simulink model "sampleModel1925"  (R2023a)
settings: Solver=VariableStepAuto  StartTime=0.0  StopTime=10.0  RelTol=1e-3
libraries: simulink x6, hdlsllib x4
settings Model: Creator=user1  LastModifiedBy=user1

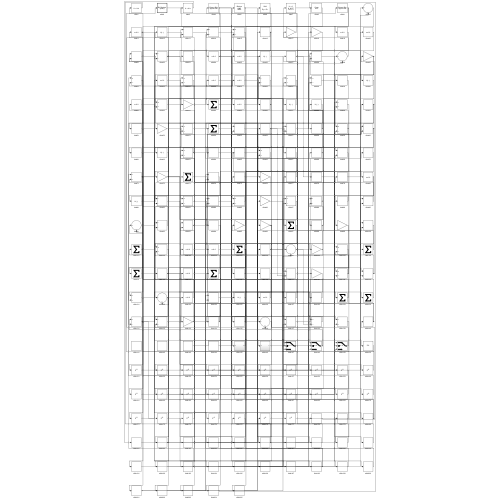
[thumbnail: Simulink's stored preview of the top-level diagram]
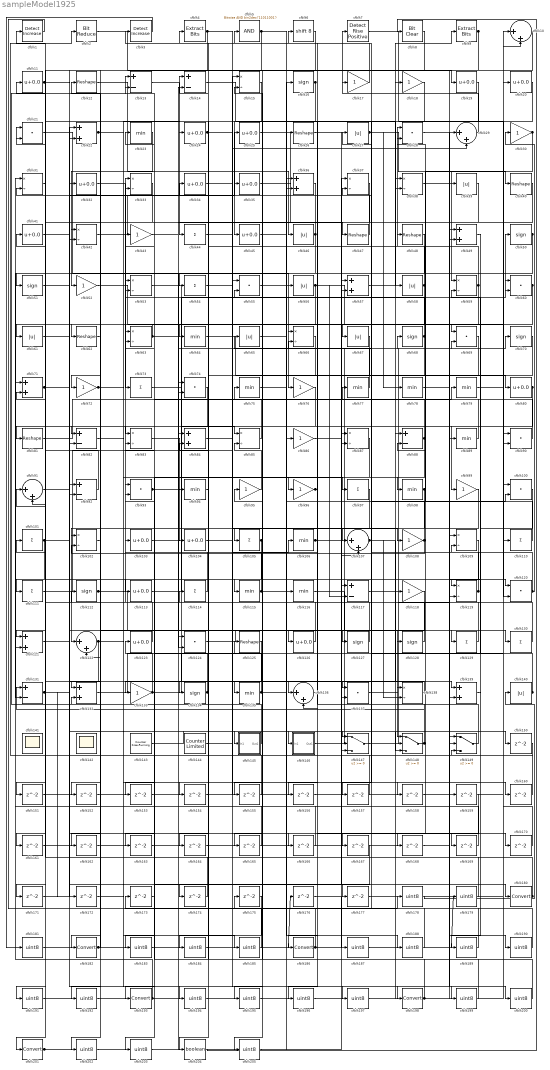
== system sampleModel1925 ==
  cfblk1 : simulink/Logic and Bit Operations/Detect Increase  vinit=0.0  OutDataTypeStr=boolean
      settings: LibrarySourceBlock=|
      | hdlsllib/Logic and Bit
      | Operations/Detect
      | Increase
  cfblk{10,29,91,107,122,136} (6 alike) : Sum  Inputs=|++
  cfblk{21,28,55,60,69,74,90,93,100,120,124,137} (12 alike) : DotProduct  OutDataTypeStr=Inherit: Inherit via internal rule
  cfblk{44,54,73,97,101,105,110..111,114,129..130} (11 alike) : Sum  Inputs=+
  cfblk{15,31,33,37..38,42,53,59,63,66,83,85,87,102,109,119,138} (17 alike) : Product  Inputs=*/  RndMeth=Zero  SaturateOnIntegerOverflow=on
  cfblk{11,19..20,24..25,32,34..35,41,45,80,103..104,113,123,126} (16 alike) : Bias  Bias=0.0  SaturateOnIntegerOverflow=off
  cfblk{23,64,75,77..79,89,94,98,106,115..116,135} (13 alike) : MinMax
  cfblk{17..18,30,43,52,72,76,86,95..96,99,108,118,133} (14 alike) : Gain
  cfblk{16,50..51,68,70,112,127..128,134} (9 alike) : Signum
  cfblk{13..14,82,88,92,117,131} (7 alike) : Sum  Inputs=+-
  cfblk{12,26,40,47..48,62,81,125} (8 alike) : Reshape
  cfblk{22,36,49,57,71,84,121,132,139} (9 alike) : Sum
  cfblk{27,39,46,56,58,61,65,67,140} (9 alike) : Abs  SaturateOnIntegerOverflow=off
  cfblk141 : Scope
      settings: Floating=on
  cfblk142 : Scope
      settings: Floating=on
  cfblk143 : hdlsllib/Sources/Counter Free-Running  NumBits=16  tsamp=-1
  cfblk144 : hdlsllib/Sources/Counter Limited  uplimit=7  tsamp=-1
  cfblk145 : Subsystem
      settings: LibrarySourceBlock=|
      | hdlsllib/Ports &
      | Subsystems/Subsystem
  cfblk146 : Subsystem
      settings: LibrarySourceBlock=|
      | hdlsllib/Ports &
      | Subsystems/Subsystem
  cfblk147 : Switch  SaturateOnIntegerOverflow=off  InputSameDT=off
  cfblk148 : Switch  SaturateOnIntegerOverflow=off  InputSameDT=off
  cfblk149 : Switch  SaturateOnIntegerOverflow=off  InputSameDT=off
  cfblk{150..177} (28 alike) : Delay  SampleTime=1
  cfblk{178..179,181,183..185,187..192,194..197,199..200,202..203,205} (21 alike) : DataTypeConversion  OutDataTypeStr=uint8  SaturateOnIntegerOverflow=off  RndMeth=Floor
  cfblk{180,182,186,193,198,201} (6 alike) : DataTypeConversion  SaturateOnIntegerOverflow=off  RndMeth=Floor
  cfblk2 : hdlsllib/Logic and Bit Operations/Bit Reduce  mode=AND
  cfblk204 : DataTypeConversion  OutDataTypeStr=boolean  SaturateOnIntegerOverflow=off  RndMeth=Floor
  cfblk3 : simulink/Logic and Bit Operations/Detect Increase  vinit=0.0  OutDataTypeStr=boolean
      settings: LibrarySourceBlock=|
      | hdlsllib/Logic and Bit
      | Operations/Detect
      | Increase
  cfblk4 : simulink/Logic and Bit Operations/Extract Bits  bitsToExtract=Upper half  numBits=8  bitIdxRange=[0 7]  outScalingMode=Preserve fixed-point scaling
      settings: LibrarySourceBlock=|
      | hdlsllib/Logic and Bit
      | Operations/Extract Bits
  cfblk5 : simulink/Logic and Bit Operations/Bitwise Operator  logicop=AND  UseBitMask=on  BitMask=bin2dec('11011001')  BitMaskRealWorld=Stored Integer
      settings: LibrarySourceBlock=|
      | hdlsllib/Logic and Bit
      | Operations/Bitwise
      | Operator
  cfblk6 : ArithShift  BitShiftNumber=8
  cfblk7 : hdlsllib/Logic and Bit Operations/Detect Rise Positive  vinit=0  OutDataTypeStr=boolean
  cfblk8 : simulink/Logic and Bit Operations/Bit Clear  iBit=0
      settings: LibrarySourceBlock=|
      | hdlsllib/Logic and Bit
      | Operations/Bit Clear
  cfblk9 : simulink/Logic and Bit Operations/Extract Bits  bitsToExtract=Upper half  numBits=8  bitIdxRange=[0 7]  outScalingMode=Preserve fixed-point scaling
      settings: LibrarySourceBlock=|
      | hdlsllib/Logic and Bit
      | Operations/Extract Bits
  wires:
  cfblk149/1 -> cfblk5/1
  cfblk53/1 -> cfblk85/1
  cfblk87/1 -> cfblk193/1
  cfblk146/1(Out1) -> cfblk68/1
  cfblk138/1 -> cfblk135/1
  cfblk23/1 -> cfblk52/1
  cfblk103/1 -> cfblk127/1
  cfblk11/1 -> cfblk170/1, cfblk171/1
  cfblk97/1 -> cfblk122/1
  cfblk81/1 -> cfblk79/1
  cfblk29/1 -> cfblk7/1
  cfblk129/1 -> cfblk33/1
  cfblk143/1 -> cfblk145/1(In1)
  cfblk88/1 -> cfblk96/1, cfblk53/2
  cfblk140/1 -> cfblk77/1, cfblk59/2
  cfblk26/1 -> cfblk180/1
  cfblk21/1 -> cfblk76/1
  cfblk106/1 -> cfblk37/1, cfblk138/1
  cfblk46/1 -> cfblk54/1, cfblk42/1
  cfblk147/1 -> cfblk70/1
  cfblk145/1(Out1) -> cfblk13/1
  cfblk116/1 -> cfblk148/1
  cfblk12/1 -> cfblk46/1
  cfblk73/1 -> cfblk137/1
  cfblk101/1 -> cfblk41/1, cfblk35/1, cfblk131/2
  cfblk32/1 -> cfblk73/1
  cfblk15/1 -> cfblk45/1
  cfblk64/1 -> cfblk109/1
  cfblk40/1 -> cfblk62/1
  cfblk65/1 -> cfblk116/1
  cfblk69/1 -> cfblk115/1
  cfblk58/1 -> cfblk28/1, cfblk102/1, cfblk27/1
  cfblk84/1 -> cfblk198/1
  cfblk102/1 -> cfblk122/2
  cfblk7/1 -> cfblk110/1
  cfblk108/1 -> cfblk37/2, cfblk102/2
  cfblk114/1 -> cfblk93/1
  cfblk89/1 -> cfblk63/1
  cfblk13/1 -> cfblk44/1
  cfblk139/1 -> cfblk2/1
  cfblk30/1 -> cfblk59/1, cfblk168/1
  cfblk85/1 -> cfblk13/2
  cfblk2/1 -> cfblk19/1
  cfblk61/1 -> cfblk147/1
  cfblk27/1 -> cfblk40/1, cfblk78/1
  cfblk48/1 -> cfblk124/2
  cfblk36/1 -> cfblk72/1
  cfblk42/1 -> cfblk25/1
  cfblk90/1 -> cfblk48/1
  cfblk113/1 -> cfblk50/1
  cfblk83/1 -> cfblk104/1
  cfblk115/1 -> cfblk14/1, cfblk100/2
  cfblk16/1 -> cfblk82/1, cfblk164/1
  cfblk111/1 -> cfblk15/1
  cfblk96/1 -> cfblk126/1, cfblk136/2
  cfblk118/1 -> cfblk182/1
  cfblk123/1 -> cfblk112/1
  cfblk39/1 -> cfblk98/1
  cfblk76/1 -> cfblk82/2
  cfblk6/1 -> cfblk105/1
  cfblk25/1 -> cfblk117/1
  cfblk131/1 -> cfblk136/1, cfblk172/1
  cfblk24/1 -> cfblk29/2, cfblk139/2
  cfblk17/1 -> cfblk3/1
  cfblk144/1 -> cfblk106/1
  cfblk59/1 -> cfblk111/1, cfblk4/1
  cfblk133/1 -> cfblk123/1, cfblk89/1
  cfblk105/1 -> cfblk151/1, cfblk152/1, cfblk195/1
  cfblk119/1 -> cfblk6/1, cfblk66/2
  cfblk4/1 -> cfblk108/1, cfblk22/2, cfblk167/1
  cfblk56/1 -> cfblk69/1, cfblk117/2, cfblk92/2
  cfblk28/1 -> cfblk130/1
  cfblk112/1 -> cfblk147/2, cfblk174/1
  cfblk50/1 -> cfblk132/1, cfblk121/2
  cfblk122/1 -> cfblk160/1, cfblk161/1
  cfblk93/1 -> cfblk39/1, cfblk53/1
  cfblk132/1 -> cfblk90/2
  cfblk47/1 -> cfblk31/2
  cfblk134/1 -> cfblk63/2, cfblk133/1
  cfblk37/1 -> cfblk147/3
  cfblk95/1 -> cfblk85/2
  cfblk60/1 -> cfblk64/1, cfblk66/1
  cfblk68/1 -> cfblk23/1, cfblk134/1
  cfblk78/1 -> cfblk120/1
  cfblk127/1 -> cfblk101/1
  cfblk20/1 -> cfblk51/1
  cfblk130/1 -> cfblk21/1
  cfblk74/1 -> cfblk201/1
  cfblk117/1 -> cfblk60/1
  cfblk45/1 -> cfblk16/1
  cfblk9/1 -> cfblk42/2, cfblk202/1
  cfblk126/1 -> cfblk114/1
  cfblk43/1 -> cfblk47/1
  cfblk72/1 -> cfblk97/1, cfblk148/3, cfblk185/1
  cfblk77/1 -> cfblk55/2
  cfblk120/1 -> cfblk109/2, cfblk30/1
  cfblk35/1 -> cfblk57/2
  cfblk124/1 -> cfblk129/1
  cfblk137/1 -> cfblk49/2
  cfblk14/1 -> cfblk58/1
  cfblk128/1 -> cfblk21/2
  cfblk92/1 -> cfblk11/1
  cfblk44/1 -> cfblk67/1
  cfblk107/1 -> cfblk139/1, cfblk138/2
  cfblk22/1 -> cfblk24/1, cfblk94/1
  cfblk54/1 -> cfblk146/1(In1)
  cfblk80/1 -> cfblk99/1, cfblk83/1
  cfblk49/1 -> cfblk119/1
  cfblk110/1 -> cfblk88/2
  cfblk121/1 -> cfblk128/1
  cfblk148/1 -> cfblk103/1, cfblk131/1
  cfblk10/1 -> cfblk149/2
  cfblk18/1 -> cfblk186/1
  cfblk57/1 -> cfblk9/1
  cfblk31/1 -> cfblk81/1
  cfblk55/1 -> cfblk80/1
  cfblk99/1 -> cfblk113/1
  cfblk5/1 -> cfblk91/2, cfblk150/1
  cfblk98/1 -> cfblk28/2, cfblk153/1
  cfblk71/1 -> cfblk22/1, cfblk121/1, cfblk199/1
  cfblk63/1 -> cfblk69/2, cfblk61/1
  cfblk52/1 -> cfblk120/2
  cfblk70/1 -> cfblk107/1
  cfblk135/1 -> cfblk15/2, cfblk60/2, cfblk83/2
  cfblk91/1 -> cfblk32/1
  cfblk79/1 -> cfblk10/2
  cfblk150/1 -> cfblk149/3
  cfblk151/1 -> cfblk55/1
  cfblk153/1 -> cfblk10/1
  cfblk82/1 -> cfblk154/1
  cfblk154/1 -> cfblk88/1
  cfblk67/1 -> cfblk155/1
  cfblk155/1 -> cfblk93/2
  cfblk136/1 -> cfblk156/1
  cfblk156/1 -> cfblk29/1
  cfblk19/1 -> cfblk157/1
  cfblk157/1 -> cfblk91/1
  cfblk86/1 -> cfblk158/1
  cfblk158/1 -> cfblk149/1
  cfblk160/1 -> cfblk57/1
  cfblk161/1 -> cfblk119/2
  cfblk62/1 -> cfblk162/1
  cfblk162/1 -> cfblk14/2
  cfblk109/1 -> cfblk163/1
  cfblk163/1 -> cfblk49/1
  cfblk164/1 -> cfblk148/2
  cfblk66/1 -> cfblk165/1
  cfblk165/1 -> cfblk71/2
  cfblk104/1 -> cfblk166/1
  cfblk166/1 -> cfblk31/1
  cfblk34/1 -> cfblk169/1
  cfblk169/1 -> cfblk124/1
  cfblk170/1 -> cfblk90/1
  cfblk171/1 -> cfblk92/1
  cfblk173/1 -> cfblk33/2
  cfblk174/1 -> cfblk12/1
  cfblk51/1 -> cfblk177/1
  cfblk177/1 -> cfblk20/1
  cfblk1/1 -> cfblk178/1
  cfblk178/1 -> cfblk140/1
  cfblk179/1 -> cfblk1/1
  cfblk180/1 -> cfblk34/1, cfblk95/1
  cfblk3/1 -> cfblk181/1
  cfblk181/1 -> cfblk26/1
  cfblk182/1 -> cfblk176/1, cfblk132/2
  cfblk125/1 -> cfblk183/1
  cfblk183/1 -> cfblk118/1
  cfblk175/1 -> cfblk184/1
  cfblk184/1 -> cfblk36/2
  cfblk185/1 -> cfblk175/1
  cfblk186/1 -> cfblk179/1, cfblk125/1, cfblk36/1
  cfblk176/1 -> cfblk187/1
  cfblk187/1 -> cfblk18/1
  cfblk75/1 -> cfblk188/1
  cfblk188/1 -> cfblk17/1
  cfblk100/1 -> cfblk189/1
  cfblk189/1 -> cfblk75/1
  cfblk38/1 -> cfblk190/1
  cfblk190/1 -> cfblk43/1
  cfblk33/1 -> cfblk191/1
  cfblk191/1 -> cfblk38/1
  cfblk152/1 -> cfblk192/1
  cfblk192/1 -> cfblk38/2
  cfblk193/1 -> cfblk100/1, cfblk71/1
  cfblk172/1 -> cfblk194/1
  cfblk194/1 -> cfblk87/1
  cfblk195/1 -> cfblk87/2
  cfblk159/1 -> cfblk196/1
  cfblk196/1 -> cfblk137/2
  cfblk41/1 -> cfblk197/1
  cfblk197/1 -> cfblk159/1
  cfblk198/1 -> cfblk173/1, cfblk65/1
  cfblk199/1 -> cfblk84/1
  cfblk168/1 -> cfblk200/1
  cfblk200/1 -> cfblk84/2
  cfblk201/1 -> cfblk107/2, cfblk56/1
  cfblk202/1 -> cfblk74/1
  cfblk167/1 -> cfblk203/1
  cfblk203/1 -> cfblk74/2
  cfblk94/1 -> cfblk204/1
  cfblk204/1 -> cfblk8/1
  cfblk8/1 -> cfblk205/1
  cfblk205/1 -> cfblk86/1

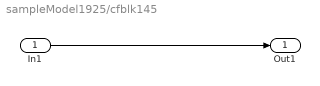
== system sampleModel1925/cfblk145 ==
  In1 : Inport
  Out1 : Outport
  wires:
  In1/1 -> Out1/1

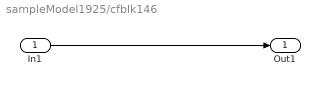
== system sampleModel1925/cfblk146 ==
  In1 : Inport
  Out1 : Outport
  wires:
  In1/1 -> Out1/1
